simulink model "propeller_characterisation"  (R2021b)
settings: Solver=VariableStepAuto  StartTime=0.0  StopTime=5  RelTol=1e-3
settings Model: Creator=cirie  LastModifiedBy=cirie

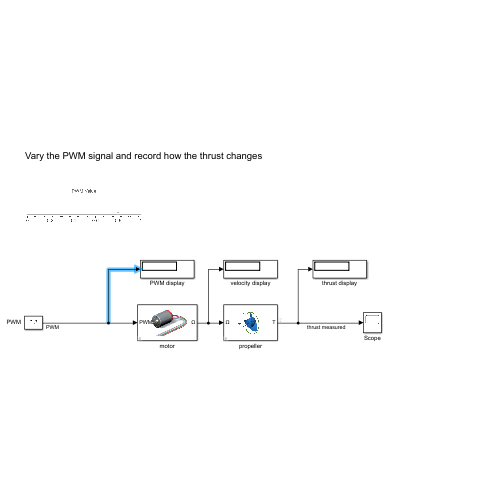
[thumbnail: Simulink's stored preview of the top-level diagram]
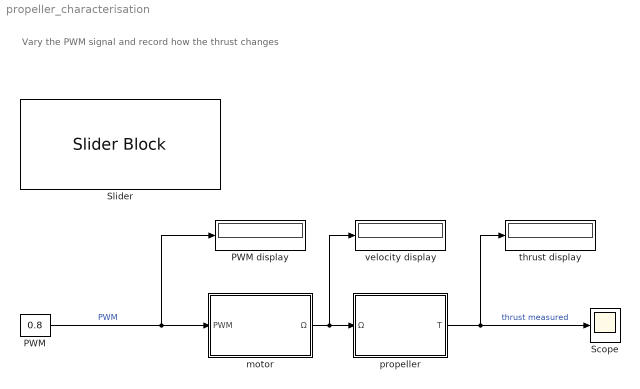
== system propeller_characterisation ==
  note: Vary the PWM signal and record how the thrust changes
  PWM : Constant  Value=0.8
  PWM display : Display
  Scope : Scope
  Slider : SliderBlock  ScaleMax=1  TickInterval=0.2
  motor : Subsystem  mask(DC Motor){J=1e-4, km=0.1, R=1, Vmax=7.2}
      mask prompts: J "Inertia, J [kgm^2]"; km "Motor constant, km [V*s/rad]"; R "Resistance, R [Ohm]"; Vmax "Maximum Voltage, Vmax [V]"
      mask help:
      | Circuit Dynamics:   PWM*Vmax == I*R + km*Ω
      | Rotor Dynamics:     J*dΩ/dt == km*I
      mask Display: image('$imagefile'); % Use "Edit Image" on toolstrip to change.
  propeller : Subsystem  mask(Propeller Model){D=0.1, kt=0.01, rho=1000}
      mask prompts: D "Propeller Diameter [m]"; kt "Thrust Coefficient"; rho "Fluid density [kg/m^3]"
      mask help: Propeller Dynamics: T = kt*rho*omega^2*D^4
      mask Display: image('$imagefile'); % Use "Edit Image" on toolstrip to change.
  thrust display : Display
  velocity display : Display
  wires:
  propeller/1(T) -> thrust display/1, Scope/1  "thrust measured"
  PWM/1 -> PWM display/1, motor/1(PWM)  "PWM"
  motor/1(Ω) -> velocity display/1, propeller/1(Ω)

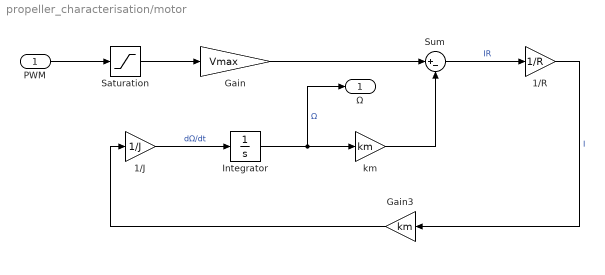
== system propeller_characterisation/motor ==
  PWM : Inport
  1/J : Gain  Gain=1/J
  1/R : Gain  Gain=1/R
  Gain : Gain  Gain=Vmax
  Gain3 : Gain  Gain=km
  Integrator : Integrator
  Saturation : Saturate  UpperLimit=1  LowerLimit=-1
  Sum : Sum  Inputs=|+-
  km : Gain  Gain=km
  Ω : Outport
  wires:
  1/J/1 -> Integrator/1  "dΩ/dt"
  Sum/1 -> 1/R/1  "IR"
  Integrator/1 -> Ω/1, km/1  "Ω"
  Gain3/1 -> 1/J/1
  km/1 -> Sum/2
  1/R/1 -> Gain3/1  "I"
  PWM/1 -> Saturation/1
  Gain/1 -> Sum/1
  Saturation/1 -> Gain/1

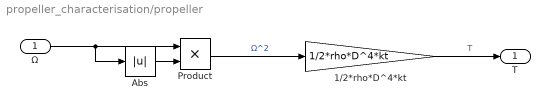
== system propeller_characterisation/propeller ==
  Ω : Inport
  1/2*rho*D^4*kt : Gain  Gain=1/2*rho*D^4*kt
  Abs : Abs
  Product : Product
  T : Outport
  wires:
  1/2*rho*D^4*kt/1 -> T/1  "T"
  Product/1 -> 1/2*rho*D^4*kt/1  "Ω^2"
  Ω/1 -> Abs/1, Product/1
  Abs/1 -> Product/2
